simulink model "Simul_dif2"  (R2021b)
settings: Solver=VariableStepAuto  StartTime=0.0  StopTime=10  RelTol=1e-3
settings Model: Creator=Alumno103  LastModifiedBy=Alumno103

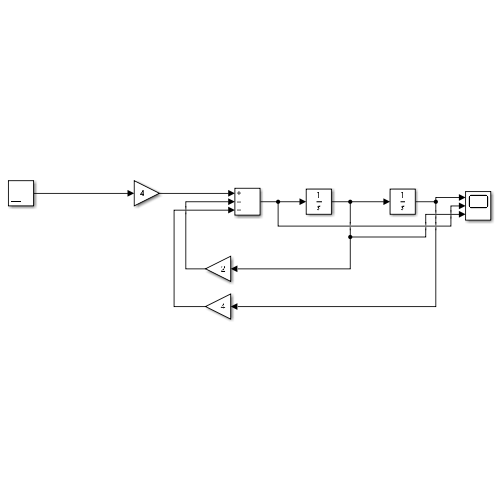
[thumbnail: Simulink's stored preview of the top-level diagram]
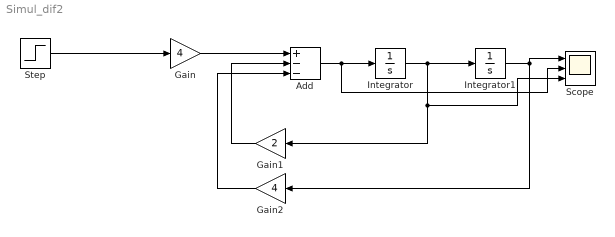
== system Simul_dif2 ==
  Add : Sum  Inputs=+--
  Gain : Gain  Gain=4
  Gain1 : Gain  Gain=2
  Gain2 : Gain  Gain=4
  Integrator : Integrator
  Integrator1 : Integrator
  Scope : Scope  NumInputPorts=3
  Step : Step  SampleTime=0
  wires:
  Step/1 -> Gain/1
  Gain/1 -> Add/1
  Add/1 -> Scope/2, Integrator/1
  Integrator/1 -> Scope/3, Gain1/1, Integrator1/1
  Integrator1/1 -> Gain2/1, Scope/1
  Gain1/1 -> Add/2
  Gain2/1 -> Add/3
